simulink model "Integration2022b_May06"  (R2022b)
settings: Solver=FixedStepAuto  StartTime=0.0  StopTime=inf  RelTol=1e-3
model workspace (MAT data in the model file):
  L = 4.165
  SL_ROS_VariableLengthArrays_MaxSizes.CommonInfo.ArrayTruncateAction = 'EmitWarning'
  SL_ROS_VariableLengthArrays_MaxSizes.MsgTypeMap = containers.Map
  SL_ROS_VariableLengthArrays_MaxSizes.MsgTypeMap.serialization.keys = {'example_interfaces/Float64MultiArray', 'std_msgs/Float32MultiArray', 'std_msgs/Float64MultiArray', 'std_msgs/Int32MultiArray'}
  SL_ROS_VariableLengthArrays_MaxSizes.MsgTypeMap.serialization.values{1}.PropertyName = 'data'
  SL_ROS_VariableLengthArrays_MaxSizes.MsgTypeMap.serialization.values{1}.DataType = 'double'
  SL_ROS_VariableLengthArrays_MaxSizes.MsgTypeMap.serialization.values{1}.MaxLength = 3
  SL_ROS_VariableLengthArrays_MaxSizes.MsgTypeMap.serialization.values{2}.PropertyName = 'data'
  SL_ROS_VariableLengthArrays_MaxSizes.MsgTypeMap.serialization.values{2}.DataType = 'single'
  SL_ROS_VariableLengthArrays_MaxSizes.MsgTypeMap.serialization.values{2}.MaxLength = 1260
  SL_ROS_VariableLengthArrays_MaxSizes.MsgTypeMap.serialization.values{3}.PropertyName = 'data'
  SL_ROS_VariableLengthArrays_MaxSizes.MsgTypeMap.serialization.values{3}.DataType = 'double'
  SL_ROS_VariableLengthArrays_MaxSizes.MsgTypeMap.serialization.values{3}.MaxLength = 1386
  SL_ROS_VariableLengthArrays_MaxSizes.MsgTypeMap.serialization.values{4}.PropertyName = 'data'
  SL_ROS_VariableLengthArrays_MaxSizes.MsgTypeMap.serialization.values{4}.DataType = 'int32'
  SL_ROS_VariableLengthArrays_MaxSizes.MsgTypeMap.serialization.values{4}.MaxLength = 3
  SL_ROS_VariableLengthArrays_MaxSizes.MsgTypeMap.serialization.uniformity = 0
  SL_ROS_VariableLengthArrays_MaxSizes.MsgTypeMap.serialization.keyType = 'char'
  SL_ROS_VariableLengthArrays_MaxSizes.MsgTypeMap.serialization.valueType = 'any'
  finalint = 0
  firstWarning = 1
  originalScenarioChecksum = '114339432DE22364D47BB28FC96DC10C'
values from neighbouring files (symbols this model uses):
  D = cross(B-A,C-A)    [HelperCalculateEgoRefPathInfo.m]
  data =     [Part_of_MCity.mat]    (also in curvedroad_Bhanu.mat; plotWPScript.m = [data, [out.x.Data(:, :, i); out.y.Data(:, :, i)]])
  x = [Vertices(Na,1) Vertices(:,1) Vertices(Nb,1)]    [HelperCalculateEgoRefPathInfo.m]    (also in HelperConvertDSPoseToSim3D.m = actor(1).Position(1); xpts.mat = [-29.9023190589 -34.2715935353 -19.4160603154 -19.4160603154)
  y = [Vertices(Na,2) Vertices(:,2) Vertices(Nb,2)]    [HelperCalculateEgoRefPathInfo.m]    (also in HelperConvertDSPoseToSim3D.m = actor(1).Position(2); VehicleOutputFcn.m = [x(1);x(2); x(3); x(4); x(5);x(6)]; ypts.mat = [-62.3254015256 -62.9079714558 -51.8391427821 -48.6350081661)
  z = zeros(1, length(interpX))    [HelperCalculateEgoRefPathInfo.m]
undefined symbols (not defined in the file or in its folder): MinVelocity, WB
libraries: ros2lib x13, mpcsigdimcheck_private x10, robotalgslib x1, mpclib x1, drivingvehiclecontroller x1, slpidlib x1
(part 1 of 5)
settings Model: Creator=akshran  LastModifiedBy=moham
settings DataIOCC: SignalLogging=off  ReturnWorkspaceOutputs=off
settings OptimizationCC: ReuseModelBlockBuffer=on  EnhancedBackFolding=on  PassReuseOutputArgsAs=Individual arguments  ZeroExternalMemoryAtStartup=off  ZeroInternalMemoryAtStartup=off  MaxStackSize=64  OptimizeBlockOrder=speed  DifferentSizesBufferReuse=on  OptimizationCustomize=off  EfficientTunableParamExpr=on
settings DebuggingCC: ParameterTunabilityLossMsg=error  UnconnectedInputMsg=warning  UnconnectedOutputMsg=warning  UnconnectedLineMsg=warning  UnderSpecifiedDimensionMsg=warning
settings HardwareCC: ProdBitPerLong=64  ProdHWDeviceType=AMD->x86-64 (Linux 64)
settings ModelReferenceCC: EnableRefExpFcnMdlSchedulingChecks=on
settings SFSimCC: MATLABDynamicMemAlloc=off
settings RTWCC: Description=Embedded Coder  SystemTargetFile=ert.tlc  HardwareBoard=Robot Operating System 2 (ROS 2)  TLCOptions="-aInlineSetEventsForThisBaseRateFcn=TLC_FALSE -aSuppressMultiTaskScheduler=TLC_FALSE  -aRateBasedStepFcn=0"  TemplateMakefile=ert_default_tmf  Toolchain=Colcon Tools  PortableWordSizes=on  TargetLang=C++  DLArmComputeVersion=19.05
settings CodeAppCC: ForceParamTrailComments=on  IgnoreCustomStorageClasses=off  OperatorAnnotations=on  SimulinkDataObjDesc=on  SFDataObjDesc=on  InsertBlockDesc=on
settings ERTTargetCC: CodeInterfacePackaging=C++ class  RootIOFormat=Structure reference
settings SettingsController: UseSoCProfilerForTargets=0

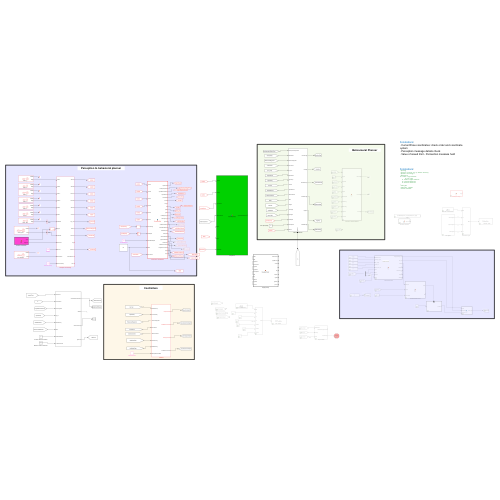
[thumbnail: Simulink's stored preview of the top-level diagram]
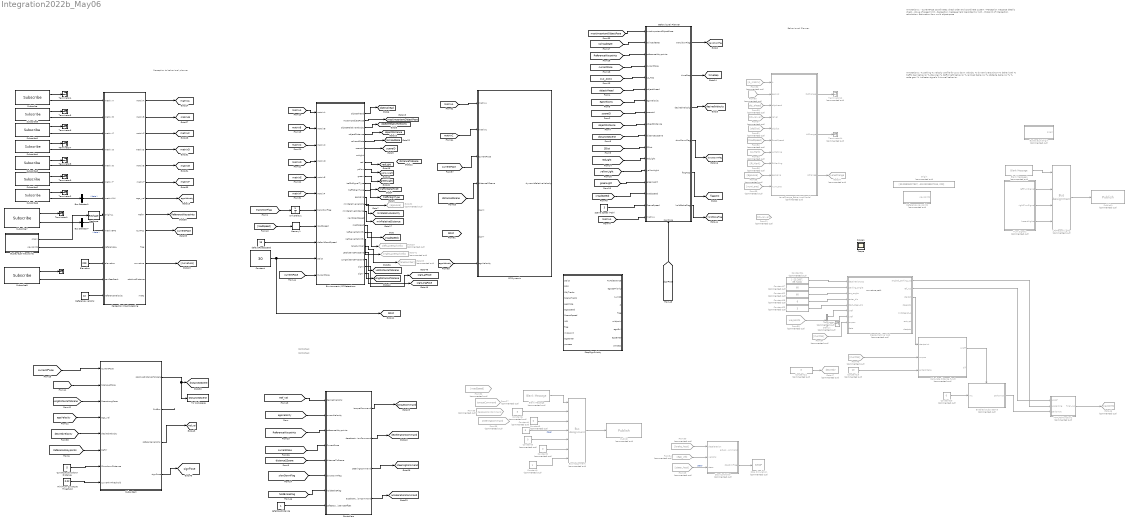
== system Integration2022b_May06 ==
  note: Annotations :
      | - CurrentPose coordinates: check order and coordinate system
      | - Perception message details check
      | - Value of speed limit - Perception message held (persistent or not)
      | - Midpoint of Intersection calculation: Estimation from multi object pose
  note: Behavioural Planner
  note: Perception to behavioral planner
  note: Controllers
  note: Controllers
  note: Annotations :
      | % parking
      | % velocity profile for up & down velocity
      | % dynamic rerouting??
      | % behavioral
      | % traffic sign behavior
      | % stop sign
      | % traffic light behavior
      | % railroad behavior
      | % obstacle behavior
      | %
      | % code gen!
      | % indicator signals
      | % tunnel behavior
  note: curvature path
  " " : Terminator
  Behavioural Planner : Subsystem
      settings: PortSchema="{\"entries\":[{\"content\":{\"sides\":[{\"content\":{\"connectorIds\":[\"In1\",\"In2\",\"In3\",\"In4\",\"In5\",\"In6\",\"In7\",\"In8\",\"In9\",\"In10\",\"In11\",\"In12\",\"In13\",\"In14\",\"In15\",\"In16\",\"In17\"]},\"type\":\"ConnectorPlacement.EquallySpacedRectSide\",\"uuid\":\"494bf481-bdc6-4ab1-b824-5f3bdb3ff01f\"},{\"content\":{\"connectorIds\":[\"Out1\",\"Out2\",\"Out3\",\"Out4\",\"Out5\",\"Out6\"],\"side\":\"RIGHT\"},\"type\":\"ConnectorPlacement.EquallySpacedRectSide\",\"uuid\":\"2468745c-f84f-4a50-a8ff-e7bb2cbe872e\"},{\"content\":{\"side\":\"TOP\"},\"type\":\"ConnectorPlacement.EquallySpacedRectSide\",\"uuid\":\"96280bc7-544f-4b45-a6db-67036c4d07c2\"},{\"content\":{\"connectorIds\":[\"In18\"],\"side\":\"BOTTOM\"},\"type\":\"ConnectorPlacement.EquallySpacedRectSide\",\"uuid\":\"4e16db0f-18f6-4a57-8589-f4480b47e9b5\"}]},\"type\":\"ConnectorPlacement.EquallySpacedConnector\",\"uuid\":\"a6b17eda-b06c-4321-9182-4c70288e8279\"}],\"packageUris\":[\"http://schema.mathworks.com/mf0/Connector/R2020b\"],\"version\":\"1.0\"}"
  Blank Message : ros2lib/Blank Message  Commented=on  messageClass=Message  entityType=std_msgs/Float64MultiArray  messageType=std_msgs/Float64MultiArray  SampleTime=0.01
      settings: LibrarySourceBlock=roslib/ROS 2/Blank Message
  Blank Message1 : ros2lib/Blank Message  Commented=on  messageClass=Message  entityType=geometry_msgs/Vector3  messageType=geometry_msgs/Vector3  SampleTime=0.01
      settings: LibrarySourceBlock=roslib/ROS 2/Blank Message
  BuckeyeLot Origin : MATLAB Function  Commented=on  TreatAsAtomicUnit=on
  BuckeyeLot Waypoints : MATLAB Function  TreatAsAtomicUnit=on
  Bus Assignment : BusAssignment  Commented=on  AssignedSignals=x,y,z,data,data,data
  Bus Selector1 : BusSelector  OutputSignals=data
  Bus Selector7 : BusSelector  OutputSignals=data
  Calculate distance func3 : MATLAB Function  Commented=on  TreatAsAtomicUnit=on
  Constant : Constant  Value=30
  Constant1 : Constant  Commented=on
  Constant17 : Constant  Commented=on  Value=60
  Constant18 : Constant  Commented=on  Value=6
  Constant19 : Constant  Commented=on  Value=10
  Constant{2..3,5,20} (4 alike) : Constant  Commented=on  Value=0
  Constant21 : Constant  Commented=on  Value=3
  Constant22 : Constant  Commented=on  Value=60
  Constant23 : Constant  Commented=on  Value=3
  Constant24 : Constant  Commented=on  Value=[ -25.2607, 39.7402]
  Constant4 : Constant  Commented=on  Value=5
  Constant6 : Constant  Commented=on  Value=5
  Controllers : Subsystem
  Create Parking Wp2 : MATLAB Function  Commented=on  TreatAsAtomicUnit=on
  Curvature Slowdown Distance : Constant  Value=5
  Demux : Demux  Commented=on  Outputs=3
  Elevation : Constant  Value=229
  Enabled Subsystem3 : Subsystem  Commented=on  TreatAsAtomicUnit=on
  Environment / SF Detections : MATLAB Function  TreatAsAtomicUnit=on
  From11 : From  Commented=on  GotoTag=obj_rel_vel  TagVisibility=global
  From27 : From  Commented=on  GotoTag=torqueCommand  TagVisibility=global
  From29 : From  Commented=on  GotoTag=steer_host  TagVisibility=global
  From30 : From  Commented=on  GotoTag=brake_host  TagVisibility=global
  From32 : From  Commented=on  GotoTag=roadSpeed
  From34 : From  Commented=on  GotoTag=ego_vel  TagVisibility=global
  From35 : From  Commented=on  GotoTag=decelerationCommand  TagVisibility=global
  From36 : From  Commented=on  GotoTag=steeringCommand  TagVisibility=global
  From37 : From  Commented=on  GotoTag=obj_rel_vel  TagVisibility=global
  From39 : From  Commented=on  GotoTag=obj_ahead  TagVisibility=global
  From49 : From  Commented=on  GotoTag=CurrPos
  From50 : From  Commented=on  GotoTag=A_matrix
  From51 : From  Commented=on  GotoTag=objDist  TagVisibility=global
  From52 : From  Commented=on  GotoTag=RoadSpeed
  From53 : From  Commented=on  GotoTag=LLMark
  From54 : From  Commented=on  GotoTag=CurrPos
  From55 : From  Commented=on  GotoTag=waypoints  TagVisibility=global
  From56 : From  Commented=on  GotoTag=RLMark
  From58 : From  Commented=on  GotoTag=EgoLane
  From59 : From  Commented=on  GotoTag=numLane
  From60 : From  Commented=on  GotoTag=ego_vel  TagVisibility=global
  Goto29 : Goto  Commented=on  GotoTag=leftLaneMarkInfo
  Goto32 : Goto  Commented=on  GotoTag=egoLane
  Goto35 : Goto  Commented=on  GotoTag=laneNumber
  Goto37 : Goto  Commented=on  GotoTag=LaneChange  TagVisibility=global
  Goto41 : Goto  Commented=on  GotoTag=rightLaneMarkInfo
  Goto46 : Goto  Commented=on  GotoTag=waypoints  TagVisibility=global
  Goto47 : Goto  Commented=on  GotoTag=desiredV  TagVisibility=global
  L/R/Hazard Lights : BusAssignment  Commented=on  AssignedSignals=x,y,z
  LaneChange_BehavioralModel : MATLAB Function  Commented=on  TreatAsAtomicUnit=on
  MATLAB Function2 : MATLAB Function  Commented=on  TreatAsAtomicUnit=on
  Memory1 : Memory  InitialCondition=15
  "Minimum Curvature Threshold " : Constant  Value=0.02
  Origin : Constant  Commented=on  Value=[39.99806227837, -83.03238507155, 229]
  Perception Pre-Processing : Subsystem
  Publish : ros2lib/Publish  Commented=on  topicSource=Select from ROS network  topic=/can_forward  messageType=geometry_msgs/Vector3  QOSHistory=Keep last  QOSDepth=1  QOSReliability=Reliable  QOSDurability=Volatile
      settings: LibrarySourceBlock=roslib/ROS 2/Publish
  Publish1 : ros2lib/Publish  Commented=on  topicSource=Specify your own  topic=/indicator_lights  messageType=geometry_msgs/Vector3  QOSHistory=Keep last  QOSDepth=1  QOSReliability=Reliable  QOSDurability=Volatile
      settings: LibrarySourceBlock=roslib/ROS 2/Publish
  Reference velocity : Constant  Value=10
  Reference waypoints : MATLAB Function  Commented=on  TreatAsAtomicUnit=on
  Reshape : Reshape  OutputDimensionality=Row vector (2-D)
  SF Dynamic : MATLAB Function  TreatAsAtomicUnit=on
  Scene Speed (Mph) : Constant  Value=3
  Stop Controller : Subsystem  Commented=on
  Stop Simulation : Stop  Commented=on
  StopSignPriority : MATLAB Function  TreatAsAtomicUnit=on
  Subscribe : ros2lib/Subscribe  topicSource=Select from ROS network  topic=/matrix_A  messageType=std_msgs/Float64MultiArray  sampleTime=-1  QOSHistory=Keep last  QOSDepth=1  QOSReliability=Reliable  QOSDurability=Volatile
      settings: LibrarySourceBlock=roslib/ROS 2/Subscribe
  Subscribe1 : ros2lib/Subscribe  topicSource=Select from ROS network  topic=/matrix_C  messageType=std_msgs/Float64MultiArray  sampleTime=-1  QOSHistory=Keep last  QOSDepth=1  QOSReliability=Reliable  QOSDurability=Volatile
      settings: LibrarySourceBlock=roslib/ROS 2/Subscribe
  Subscribe2 : ros2lib/Subscribe  topicSource=Select from ROS network  topic=/matrix_F  messageType=std_msgs/Float64MultiArray  sampleTime=-1  QOSHistory=Keep last  QOSDepth=1  QOSReliability=Reliable  QOSDurability=Volatile
      settings: LibrarySourceBlock=roslib/ROS 2/Subscribe
  Subscribe3 : ros2lib/Subscribe  topicSource=Select from ROS network  topic=/matrix_E  messageType=std_msgs/Float64MultiArray  sampleTime=-1  QOSHistory=Keep last  QOSDepth=1  QOSReliability=Reliable  QOSDurability=Volatile
      settings: LibrarySourceBlock=roslib/ROS 2/Subscribe
  Subscribe4 : ros2lib/Subscribe  topicSource=Select from ROS network  topic=/matrix_D  messageType=std_msgs/Float64MultiArray  sampleTime=-1  QOSHistory=Keep last  QOSDepth=1  QOSReliability=Reliable  QOSDurability=Volatile
      settings: LibrarySourceBlock=roslib/ROS 2/Subscribe
  Subscribe5 : ros2lib/Subscribe  topicSource=Select from ROS network  topic=/matrix_B  messageType=std_msgs/Float64MultiArray  sampleTime=-1  QOSHistory=Keep last  QOSDepth=1  QOSReliability=Reliable  QOSDurability=Volatile
      settings: LibrarySourceBlock=roslib/ROS 2/Subscribe
  Subscribe6 : ros2lib/Subscribe  topicSource=Select from ROS network  topic=/matrix_IMU  messageType=std_msgs/Float64MultiArray  sampleTime=-1  QOSHistory=Keep all  QOSDepth=1  QOSReliability=Reliable  QOSDurability=Volatile
      settings: LibrarySourceBlock=roslib/ROS 2/Subscribe
  Subscribe7 : ros2lib/Subscribe  topicSource=Specify your own  topic=/matrix_GPS  messageType=std_msgs/Float64MultiArray  sampleTime=-1  QOSHistory=Keep all  QOSDepth=1  QOSReliability=Reliable  QOSDurability=Volatile
      settings: LibrarySourceBlock=roslib/ROS 2/Subscribe
  Subscribe9 : ros2lib/Subscribe  topicSource=Specify your own  topic=/can_feedback  messageType=geometry_msgs/Vector3  sampleTime=-1  QOSHistory=Keep all  QOSDepth=1  QOSReliability=Reliable  QOSDurability=Volatile
      settings: LibrarySourceBlock=roslib/ROS 2/Subscribe
  Subsystem : Subsystem
  Terminator : Terminator  Commented=on
  Terminator{1..2,4..9} (8 alike) : Terminator
  Terminator12 : Terminator  Commented=on
  Terminator14 : Terminator  Commented=on
  To Workspace : ToWorkspace  VariableName=Distance2Scene  SaveFormat=Structure With Time  SampleTime=-1
  Turn Signals : Subsystem  Commented=on
  Unit Delay1 : UnitDelay  SampleTime=0.01  HasFrameUpgradeWarning=on
  defaultRoadSpeed : Constant  Value=15
  safeStopDistance : Constant
  Scope : Scope
  Scope1 : Scope
  tag scope: LatDistanceToScene=global, LongDistanceToScene=global, Ref_Vel=global, ReferenceWaypoints=global, SDist=global, accelerationCommand=global, currentPose=global, decelerationCommand=global, desiredVelocity=global, distance2Scene=global, distanceToScene=global, egoVelocity=global, flagACC=global, greenLight=global, holdBrakeFlag=global, matrixA=global, matrixB=global, matrixC=global, matrixD=global, matrixE=global, matrixF=global, minRelativeDistance=global, minRelativeVelocity=global, mostImportantObjectPose=global, objectAhead=global, objectDistance=global, objectRelativeVelocity=global, railroadGate=global, redLight=global, sceneID=global, signLatPose=global, signLongPose=global, signPose=global, slowDownFlag=global, steeringCommand=global, timeGap=global, torqueCommand=global, trafficSignType=global, trafficSignalType=global, transitionFlag=global, yellowLight=global
  wires:
  [transitionFlag] -> Unit Delay1/1
  [objectAhead] -> Behavioural Planner/6(objectAhead)
  [egoVelocity] -> Behavioural Planner/7(egoVelocity)
  [objectDistance] -> Behavioural Planner/9(objectDistance)
  [SDist] -> Behavioural Planner/11(SDist)
  Behavioural Planner/5(flagACC) -> [flagACC]
  Behavioural Planner/1(transitionFlag) -> [transitionFlag]
  Behavioural Planner/2(timeGap) -> [timeGap]
  Behavioural Planner/3(desiredVelocity) -> [desiredVelocity]
  Behavioural Planner/4(slowDownFlag) -> [slowDownFlag]
  [LC_ACC] -> Behavioural Planner/5(LC_ACC)
  [redLight] -> Behavioural Planner/12(redLight)
  [yellowLight] -> Behavioural Planner/13(yellowLight)
  [greenLight] -> Behavioural Planner/14(greenLight)
  [railroadGate] -> Behavioural Planner/2(railroadGate)
  [currentPose] -> Behavioural Planner/4(currentPose)
  From50/1 -> LaneChange_BehavioralModel/1(A)
  From39/1 -> LaneChange_BehavioralModel/3(objahead)
  From37/1 -> LaneChange_BehavioralModel/4(relvel)
  From51/1 -> LaneChange_BehavioralModel/5(objdist)
  From52/1 -> LaneChange_BehavioralModel/6(RoadSpeed)
  From53/1 -> LaneChange_BehavioralModel/7(LLMarking)
  From56/1 -> LaneChange_BehavioralModel/8(RLMarking)
  From58/1 -> LaneChange_BehavioralModel/9(egoLane)
  From59/1 -> LaneChange_BehavioralModel/10(numLane)
  From60/1 -> LaneChange_BehavioralModel/2(egovel)
  LaneChange_BehavioralModel/1(RLChange) -> Terminator12/1
  LaneChange_BehavioralModel/2(LLChange) -> Terminator14/1
  LaneChange_BehavioralModel/3(LChange) -> Goto37/1
  Subscribe2/1 -> Terminator9/1
  Subscribe5/1 -> Terminator5/1
  Subscribe1/1 -> Terminator6/1
  Subscribe3/1 -> Terminator8/1
  Subscribe/1 -> Terminator4/1
  Subscribe4/1 -> Terminator7/1
  Subscribe9/1 -> " "/1
  Perception Pre-Processing/6(matrixF) -> [matrixF]
  Perception Pre-Processing/4(matrixD) -> [matrixD]
  Perception Pre-Processing/1(matrixA) -> [matrixA]
  Perception Pre-Processing/2(matrixB) -> [matrixB]
  Subscribe/2 -> Perception Pre-Processing/1(matrix A)
  Subscribe5/2 -> Perception Pre-Processing/2(matrix B)
  Subscribe1/2 -> Perception Pre-Processing/3(matrix C)
  Subscribe4/2 -> Perception Pre-Processing/4(matrix D)
  Subscribe3/2 -> Perception Pre-Processing/5(matrix E)
  Subscribe2/2 -> Perception Pre-Processing/6(matrix F)
  BuckeyeLot Waypoints/1(origin) -> Reshape/1
  BuckeyeLot Waypoints/2(waypoints) -> Perception Pre-Processing/10(referenceLL)
  Elevation/1 -> Perception Pre-Processing/11(elevation)
  Subscribe9/2 -> Perception Pre-Processing/12(canFeedback)
  Reference velocity/1 -> Perception Pre-Processing/13(referenceVelocity)
  Perception Pre-Processing/7(ego_vel) -> [egoVelocity]
  Perception Pre-Processing/8(RefXY) -> [ReferenceWaypoints]
  Perception Pre-Processing/9(CurrPos) -> [currentPose]
  Perception Pre-Processing/11(curvature) -> [curvature]
  Perception Pre-Processing/3(matrixC) -> [matrixC]
  [matrixA] -> Environment / SF Detections/1(matrixA)
  [matrixB] -> Environment / SF Detections/2(matrixB)
  [matrixC] -> Environment / SF Detections/3(matrixC)
  [matrixD] -> Environment / SF Detections/4(matrixD)
  [matrixE] -> Environment / SF Detections/5(matrixE)
  Unit Delay1/1 -> Environment / SF Detections/7(transitionFlag)
  Constant/1 -> [SDist], Environment / SF Detections/10(SDist)
  Controllers/4(accelerationCommand) -> [accelerationCommand]
  Controllers/1(torqueCommand) -> [torqueCommand]
  Controllers/3(steeringCommand) -> [steeringCommand]
  [ReferenceWaypoints] -> Controllers/3(referenceWaypoints)
  [currentPose] -> Controllers/4(CurrentPose)
  [egoVelocity] -> Controllers/2(currentVelocity)
  Controllers/2(decelerationCommand) -> [decelerationCommand]
  [slowDownFlag] -> Controllers/6(slowDownFlag)
  Bus Assignment/1 -> Publish/1
  Constant6/1 -> Bus Assignment/2
  Blank Message/1 -> Bus Assignment/1
  Constant5/1 -> Bus Assignment/3
  From30/1 -> Stop Controller/1(deceleration)
  From34/1 -> Stop Controller/2(velocity)
  From29/1 -> Stop Controller/3(steer)  "steer"
  Stop Controller/2(stopSimFlag) -> Stop Simulation/1
  Turn Signals/1(leftTurnSignal) -> L/R/Hazard Lights/2
  Turn Signals/3(hazardLights) -> L/R/Hazard Lights/4
  Turn Signals/2(rightTurnSignal) -> L/R/Hazard Lights/3
  L/R/Hazard Lights/1 -> Publish1/1
  Blank Message1/1 -> L/R/Hazard Lights/1
  [ReferenceWaypoints] -> Behavioural Planner/3(referenceWaypoints)
  Environment / SF Detections/1(objectAhead) -> [objectAhead]
  Environment / SF Detections/2(mostImpObjectPose) -> [mostImportantObjectPose]
  Environment / SF Detections/3(objectRelativeVelocity) -> [objectRelativeVelocity]
  Environment / SF Detections/4(objectDistance) -> [objectDistance]
  Environment / SF Detections/5(railroadGate) -> [railroadGate]
  Environment / SF Detections/6(sceneId) -> [sceneID]
  Environment / SF Detections/8(red) -> [redLight]
  Environment / SF Detections/9(yellow) -> [yellowLight]
  Environment / SF Detections/10(green) -> [greenLight]
  Environment / SF Detections/11(trafficSignalType) -> [trafficSignalType]
  Environment / SF Detections/12(trafficSignType) -> [trafficSignType]
  Environment / SF Detections/13(egoLane) -> Goto32/1
  Environment / SF Detections/14(minRelativeVelocity) -> [minRelativeVelocity]
  Environment / SF Detections/15(minRelativeDistance) -> [minRelativeDistance]
  Environment / SF Detections/20(laneNumber) -> Goto35/1
  Environment / SF Detections/18(leftLaneMarkInfo) -> Goto29/1
  Environment / SF Detections/19(rightLaneMarkInfo) -> Goto41/1
  [matrixF] -> Environment / SF Detections/6(matrixF)
  safeStopDistance/1 -> Controllers/8(safeStopDistanceOffset)
  Scene Speed (Mph)/1 -> Behavioural Planner/16(SceneSpeed)
  Environment / SF Detections/17(roadSpeed) -> [roadSpeed]
  [mostImportantObjectPose] -> Behavioural Planner/1(mostImportantObjectPose)
  Reshape/1 -> Perception Pre-Processing/8(originLL)
  Subscribe7/2 -> Bus Selector7/1
  Bus Selector7/1 -> Perception Pre-Processing/9(matrixGPS)  "<data>"
  Bus Selector1/1 -> Perception Pre-Processing/7(matrixIMU)  "<data>"
  Subscribe7/1 -> Terminator1/1
  Subscribe6/1 -> Terminator2/1
  Subscribe6/2 -> Bus Selector1/1
  [distance2Scene] -> Behavioural Planner/10(distance2Scene)
  [distance2Scene] -> Controllers/5(distanceToScene)
  Constant4/1 -> Bus Assignment/4  "steer"
  [sceneID] -> Behavioural Planner/8(sceneId)
  [egoVelocity] -> Subsystem/4(ego_vel)
  [desiredVelocity] -> Subsystem/5(desiredVelocity)
  [ReferenceWaypoints] -> Subsystem/6(RefXY)
  Curvature Slowdown Distance/1 -> Subsystem/7(SlowdownDistance)
  "Minimum Curvature Threshold "/1 -> Subsystem/8(curveMinThreshold)
  Subsystem/1(relativeDistanceToScene) -> To Workspace/1, [distance2Scene]
  [currentPose] -> Subsystem/1(CurrentPose)
  Environment / SF Detections/21(LatDistanceToScene) -> [LatDistanceToScene]
  Environment / SF Detections/22(LongDistanceToScene) -> [LongDistanceToScene]
  [LatDistanceToScene] -> Subsystem/2(SceneLatPose)
  [LongDistanceToScene] -> Subsystem/3(SceneLongPose)
  Subsystem/3(referenceVelocity) -> [Ref_Vel]
  [Ref_Vel] -> Controllers/1(desiredVelocity)
  Perception Pre-Processing/5(matrixE) -> [matrixE]
  [currentPose] -> Environment / SF Detections/11(CurrentPose)
  [roadSpeed] -> Behavioural Planner/15(roadSpeed)
  Behavioural Planner/6(holdBrakeFlag) -> [holdBrakeFlag]
  [holdBrakeFlag] -> Controllers/7(holdBrakeFlag)
  [matrixA] -> Behavioural Planner/17(matrixA)
  [signPose] -> Behavioural Planner/18(signPose)
  Subsystem/4(signPose) -> [signPose]
  defaultRoadSpeed/1 -> Environment / SF Detections/9(defaultRoadSpeed)
  Constant20/1 -> Enabled Subsystem3/1(In1)
  Constant18/1 -> Create Parking Wp2/4(enter_dis)
  Create Parking Wp2/2(ref_wp) -> MATLAB Function2/1(wpref)
  Constant19/1 -> Calculate distance func3/3(entercriteria)
  Constant23/1 -> Create Parking Wp2/5(start_steer_dis)
  From49/1 -> Calculate distance func3/2(curpos)
  Constant17/1 -> Create Parking Wp2/2(parking_angle)
  Calculate distance func3/1(onoff) -> Enabled Subsystem3/Enable
  Constant22/1 -> Create Parking Wp2/3(arc_angle)
  Constant21/1 -> Goto47/1
  Enabled Subsystem3/1(parkornot) -> MATLAB Function2/3(parkornot)
  Constant24/1 -> Create Parking Wp2/1(destinationpos)
  Create Parking Wp2/1(angled_parking_wp) -> MATLAB Function2/2(wpparking)
  MATLAB Function2/1(final_wp) -> Goto46/1
  Create Parking Wp2/3(startpt) -> Calculate distance func3/1(startpoint)
  From54/1 -> Create Parking Wp2/8(curpos)
  From55/1 -> Demux/1
  Demux/1 -> Create Parking Wp2/6(xref)
  Demux/2 -> Create Parking Wp2/7(yref)
  Demux/3 -> Terminator/1
  Constant1/1 -> Bus Assignment/7
  Constant2/1 -> Bus Assignment/6
  Constant3/1 -> Bus Assignment/5
  [roadSpeed] -> Memory1/1
  Memory1/1 -> Environment / SF Detections/8("roadSpeed ")
  [currentPose] -> SF Dynamic/3(CurrentPose)
  [matrixA] -> SF Dynamic/1(matrixA)
  [distance2Scene] -> SF Dynamic/4(distance2Scene)
  Subsystem/2(OutBus) -> ?
  [matrixC] -> SF Dynamic/2(matrixC)
  Environment / SF Detections/23(signX) -> [signLatPose]
  Environment / SF Detections/24(signY) -> [signLongPose]
  [egoVelocity] -> SF Dynamic/7(egoVelocity)

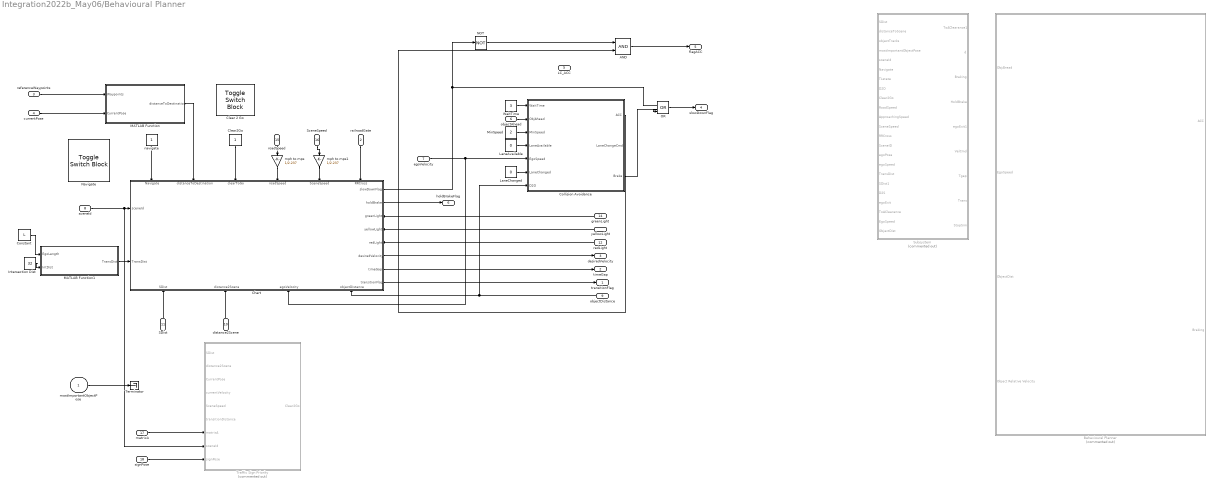
== system Integration2022b_May06/Behavioural Planner ==
  mostImportantObjectPose : Inport
  railroadGate : Inport  Port=2
  referenceWaypoints : Inport  Port=3
  currentPose : Inport  Port=4
  LC_ACC : Inport  Port=5
  objectAhead : Inport  Port=6
  egoVelocity : Inport  Port=7
  sceneId : Inport  Port=8
  objectDistance : Inport  Port=9
  distance2Scene : Inport  Port=10
  SDist : Inport  Port=11
  redLight : Inport  Port=12
  yellowLight : Inport  Port=13
  greenLight : Inport  Port=14
  roadSpeed : Inport  Port=15
  SceneSpeed : Inport  Port=16
  matrixA : Inport  Port=17
  signPose : Inport  Port=18
  AND : Logic  IconShape=distinctive  AllPortsSameDT=off  OutDataTypeStr=fixdt(1,16)
  Behavioural Planner : Subsystem  Commented=on
  Chart : Stateflow chart  TreatAsAtomicUnit=on
      settings: PortSchema="{\"entries\":[{\"content\":{\"sides\":[{\"content\":{\"connectorIds\":[\"In14\",\"In4\"]},\"type\":\"ConnectorPlacement.EquallySpacedRectSide\",\"uuid\":\"81aca70f-0947-49fb-b60a-be241e44193b\"},{\"content\":{\"connectorIds\":[\"Out4\",\"Out5\",\"In1\",\"In2\",\"In3\",\"Out1\",\"Out2\",\"Out3\"],\"side\":\"RIGHT\"},\"type\":\"ConnectorPlacement.EquallySpacedRectSide\",\"uuid\":\"e7b9645e-3711-4964-ac9b-0199dd335e99\"},{\"content\":{\"connectorIds\":[\"In15\",\"In11\",\"In12\",\"In13\",\"In7\",\"In9\"],\"side\":\"TOP\"},\"type\":\"ConnectorPlacement.EquallySpacedRectSide\",\"uuid\":\"6876f024-944b-4540-9404-d68f37763657\"},{\"content\":{\"connectorIds\":[\"In8\",\"In10\",\"In5\",\"In6\"],\"side\":\"BOTTOM\"},\"type\":\"ConnectorPlacement.EquallySpacedRectSide\",\"uuid\":\"44acab73-cdde-4edf-95df-27422644ccab\"}]},\"type\":\"ConnectorPlacement.EquallySpacedConnector\",\"uuid\":\"d2c31c01-e447-43db-8d2b-8b98a0ca291a\"}],\"packageUris\":[\"http://schema.mathworks.com/mf0/Connector/R2020b\"],\"version\":\"1.0\"}"
  Clear 2 Go : ToggleSwitchBlock
      settings: Values={{'Off', 'On'}, [0 1]}
  Clear2Go : Constant
  Collision Avoidance : Stateflow chart  TreatAsAtomicUnit=on
  Constant : Constant  Value=L
  Intersection Dist : Constant  Value=32
  LaneAvailable : Constant  Value=0
  LaneChanged : Constant  Value=0
  MATLAB Function : MATLAB Function  TreatAsAtomicUnit=on
  MATLAB Function1 : MATLAB Function  TreatAsAtomicUnit=on
  MinSpeed : Constant  Value=2
  NOT : Logic  Operator=NOT  IconShape=distinctive  AllPortsSameDT=off  OutDataTypeStr=boolean
  Navigate : ToggleSwitchBlock
      settings: Values={{'Off', 'On'}, [0 1]}
  OR : Logic  Operator=OR  IconShape=distinctive  AllPortsSameDT=off  OutDataTypeStr=boolean
  Subsystem : Subsystem  Commented=on
  Terminator : Terminator
  Traffic Sign Priority : MATLAB Function  Commented=on  TreatAsAtomicUnit=on
  WaitTime : Constant  Value=3
  mph to mps : Gain  Gain=1/2.237
  mph to mps1 : Gain  Gain=1/2.237
  navigate : Constant
  transitionFlag : Outport
  timeGap : Outport  Port=2
  desiredVelocity : Outport  Port=3
  slowDownFlag : Outport  Port=4
  flagACC : Outport  Port=5
  holdBrakeFlag : Outport  Port=6
  wires:
  Clear2Go/1 -> Chart/12(clearToGo)
  objectDistance/1 -> Collision Avoidance/7(D2O), Chart/6(objectDistance)
  WaitTime/1 -> Collision Avoidance/1(WaitTime)
  navigate/1 -> Chart/15(Navigate)
  egoVelocity/1 -> Collision Avoidance/5(EgoSpeed), Chart/5(egoVelocity)
  LaneAvailable/1 -> Collision Avoidance/4(LaneAvailable)
  currentPose/1 -> MATLAB Function/2(CurrentPose)
  MinSpeed/1 -> Collision Avoidance/3(MinSpeed)
  LaneChanged/1 -> Collision Avoidance/6(LaneChanged)
  objectAhead/1 -> Collision Avoidance/2(ObjAhead)
  MATLAB Function/1(distanceToDestination) -> Chart/11(distanceToDestination)
  Chart/3(transitionFlag) -> transitionFlag/1
  Chart/1(desiredVelocity) -> desiredVelocity/1
  SDist/1 -> Chart/8(SDist)
  distance2Scene/1 -> Chart/10(distance2Scene)
  Chart/2(timeGap) -> timeGap/1
  Collision Avoidance/1(ACC) -> AND/2
  NOT/1 -> AND/1
  Chart/4(slowDownFlag) -> NOT/1, OR/1
  OR/1 -> slowDownFlag/1
  Collision Avoidance/3(Brake) -> OR/2
  Constant/1 -> MATLAB Function1/1(EgoLength)
  Intersection Dist/1 -> MATLAB Function1/2(IntDist)
  MATLAB Function1/1(TransDist) -> Chart/4(TransDist)
  yellowLight/1 -> Chart/2(yellowLight)
  redLight/1 -> Chart/3(redLight)
  railroadGate/1 -> Chart/9(RRCross)
  referenceWaypoints/1 -> MATLAB Function/1(Waypoints)
  mph to mps/1 -> Chart/13(roadSpeed)
  roadSpeed/1 -> mph to mps/1
  greenLight/1 -> Chart/1(greenLight)
  AND/1 -> flagACC/1
  SceneSpeed/1 -> mph to mps1/1
  mph to mps1/1 -> Chart/7(SceneSpeed)
  mostImportantObjectPose/1 -> Terminator/1
  Chart/5(holdBrake) -> holdBrakeFlag/1
  matrixA/1 -> Traffic Sign Priority/7(matrixA)
  signPose/1 -> Traffic Sign Priority/9(signPose)
  sceneId/1 -> Traffic Sign Priority/8(sceneId), Chart/14(sceneId)

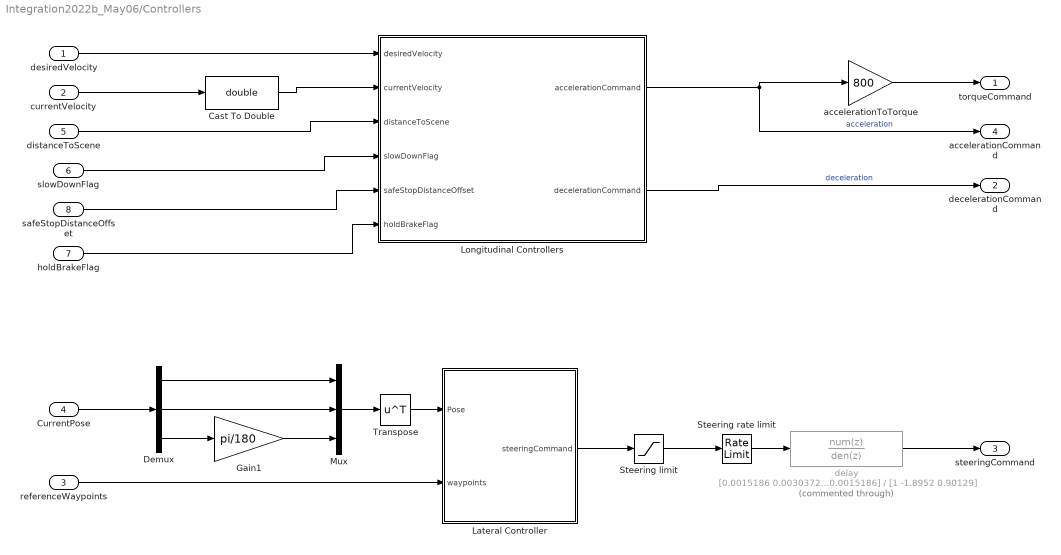
== system Integration2022b_May06/Controllers ==
  desiredVelocity : Inport
  currentVelocity : Inport  Port=2
  referenceWaypoints : Inport  Port=3
  CurrentPose : Inport  Port=4
  distanceToScene : Inport  Port=5
  slowDownFlag : Inport  Port=6
  holdBrakeFlag : Inport  Port=7
  safeStopDistanceOffset : Inport  Port=8
  Cast To Double : DataTypeConversion  OutDataTypeStr=double  SaturateOnIntegerOverflow=off  RndMeth=Floor
  Demux : Demux  Outputs=3
  Gain1 : Gain  Gain=pi/180
  Lateral Controller : Subsystem
  Longitudinal Controllers : Subsystem
  Mux : Mux  Inputs=3
  Steering limit : Saturate  UpperLimit=540  LowerLimit=-540  LinearizeAsGain=off
  Steering rate limit : RateLimiter  RisingSlewLimit=600  FallingSlewLimit=-600  SampleTimeMode=inherited
  Transpose : Math  Operator=transpose  SignedPower=on
  accelerationToTorque : Gain  Gain=800
  delay : DiscreteTransferFcn  Commented=through  Numerator=[0.0015186 0.0030372 0.0015186]  Denominator=[1 -1.8952 0.90129]  SampleTime=0.01
  torqueCommand : Outport
  decelerationCommand : Outport  Port=2
  steeringCommand : Outport  Port=3
  accelerationCommand : Outport  Port=4
  wires:
  desiredVelocity/1 -> Longitudinal Controllers/1(desiredVelocity)
  Longitudinal Controllers/2(decelerationCommand) -> decelerationCommand/1  "deceleration"
  Longitudinal Controllers/1(accelerationCommand) -> accelerationToTorque/1, accelerationCommand/1  "acceleration"
  currentVelocity/1 -> Cast To Double/1
  CurrentPose/1 -> Demux/1
  referenceWaypoints/1 -> Lateral Controller/2(waypoints)
  Cast To Double/1 -> Longitudinal Controllers/2(currentVelocity)
  Steering limit/1 -> Steering rate limit/1
  Lateral Controller/1(steeringCommand) -> Steering limit/1
  delay/1 -> steeringCommand/1
  accelerationToTorque/1 -> torqueCommand/1
  distanceToScene/1 -> Longitudinal Controllers/3(distanceToScene)
  slowDownFlag/1 -> Longitudinal Controllers/4(slowDownFlag)
  Mux/1 -> Transpose/1
  Demux/3 -> Gain1/1
  Demux/2 -> Mux/2
  Demux/1 -> Mux/1
  Transpose/1 -> Lateral Controller/1(Pose)
  Gain1/1 -> Mux/3
  safeStopDistanceOffset/1 -> Longitudinal Controllers/5(safeStopDistanceOffset)
  Steering rate limit/1 -> delay/1
  holdBrakeFlag/1 -> Longitudinal Controllers/6(holdBrakeFlag)

== system Integration2022b_May06/Enabled Subsystem3 ==
  In1 : Inport
  Enable : EnablePort
  Constant : Constant
  Sum : Sum
  parkornot : Outport
  wires:
  In1/1 -> Sum/1
  Constant/1 -> Sum/2
  Sum/1 -> parkornot/1

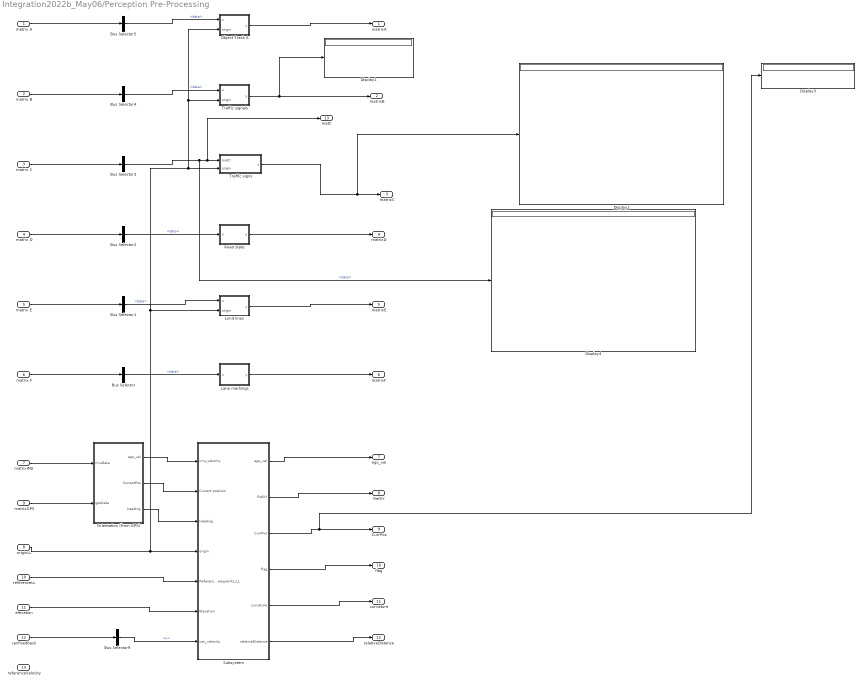
== system Integration2022b_May06/Perception Pre-Processing ==
  matrix A : Inport
  matrix B : Inport  Port=2
  matrix C : Inport  Port=3
  matrix D : Inport  Port=4
  matrix E : Inport  Port=5
  matrix F : Inport  Port=6
  matrixIMU : Inport  Port=7
  originLL : Inport  Port=8
  matrixGPS : Inport  Port=9
  referenceLL : Inport  Port=10
  elevation : Inport  Port=11
  canFeedback : Inport  Port=12
  referenceVelocity : Inport  Port=13
  Bus Selector{,1..5} (6 alike) : BusSelector  OutputSignals=data
  Bus Selector9 : BusSelector  OutputSignals=x
  Display{1..4} (4 alike) : Display
  Lane markings : MATLAB Function  TreatAsAtomicUnit=on
  Limit lines : MATLAB Function  TreatAsAtomicUnit=on
  Object Track A : MATLAB Function  TreatAsAtomicUnit=on
  Orientation (from GPS) : MATLAB Function  TreatAsAtomicUnit=on
  Road state : MATLAB Function  TreatAsAtomicUnit=on
  Subsystem : Subsystem
  Traffic signals : MATLAB Function  TreatAsAtomicUnit=on
  Traffic signs : MATLAB Function  TreatAsAtomicUnit=on
  matrixA : Outport
  matrixB : Outport  Port=2
  matrixC : Outport  Port=3
  matrixD : Outport  Port=4
  matrixE : Outport  Port=5
  matrixF : Outport  Port=6
  ego_vel : Outport  Port=7
  RefXY : Outport  Port=8
  CurrPos : Outport  Port=9
  flag : Outport  Port=10
  curvature : Outport  Port=11
  relativeDistance : Outport  Port=12
  matC : Outport  Port=13
  wires:
  Bus Selector2/1 -> Road state/1(u)  "<data>"
  matrixIMU/1 -> Orientation (from GPS)/1(imuData)
  Bus Selector1/1 -> Limit lines/1(u)  "<data>"
  Bus Selector4/1 -> Traffic signals/1(u)  "<data>"
  Bus Selector9/1 -> Subsystem/7(can_velocity)  "<x>"
  Bus Selector5/1 -> Object Track A/1(u)  "<data>"
  Orientation (from GPS)/1(ego_vel) -> Subsystem/1(imu_velocity)
  Road state/1(y) -> matrixD/1
  matrix A/1 -> Bus Selector5/1
  Bus Selector3/1 -> Display4/1, matC/1, Traffic signs/1(matC)  "<data>"
  matrix E/1 -> Bus Selector1/1
  Bus Selector/1 -> Lane markings/1(u)  "<data>"
  Orientation (from GPS)/2(CurrentPos) -> Subsystem/2(Current position)
  Limit lines/1(y) -> matrixE/1
  Orientation (from GPS)/3(heading) -> Subsystem/3(Heading)
  Object Track A/1(y) -> matrixA/1
  matrix D/1 -> Bus Selector2/1
  matrix C/1 -> Bus Selector3/1
  matrix B/1 -> Bus Selector4/1
  Subsystem/4(flag) -> flag/1
  matrix F/1 -> Bus Selector/1
  canFeedback/1 -> Bus Selector9/1
  referenceLL/1 -> Subsystem/5(Reference_waypoints_LL)
  elevation/1 -> Subsystem/6(Elevation)
  Subsystem/3(CurrPos) -> CurrPos/1, Display3/1
  Subsystem/1(ego_vel) -> ego_vel/1
  Lane markings/1(y) -> matrixF/1
  Subsystem/2(RefXY) -> RefXY/1
  Subsystem/5(curvature) -> curvature/1
  matrixGPS/1 -> Orientation (from GPS)/2(gpsData)
  Subsystem/6(relativeDistance) -> relativeDistance/1
  originLL/1 -> Limit lines/2(origin), Object Track A/2(origin), Traffic signals/2(origin), Traffic signs/2(origin), Subsystem/4(origin)
  Traffic signals/1(y) -> Display1/1, matrixB/1
  Traffic signs/1(y) -> Display2/1, matrixC/1

== system Integration2022b_May06/Stop Controller ==
  deceleration : Inport
  velocity : Inport  Port=2
  steer : Inport  Port=3
  Brake Safety : MATLAB Function  TreatAsAtomicUnit=on
  MATLAB Function5 : MATLAB Function  TreatAsAtomicUnit=on
  Steer Safety : MATLAB Function  TreatAsAtomicUnit=on
  actualSteeringCommand : Outport
  stopSimFlag : Outport  Port=2
  wires:
  Brake Safety/1(actualDeceleration) -> MATLAB Function5/2(braking)
  [accelerationCommand] -> MATLAB Function5/1(acceleration)
  steer/1 -> Steer Safety/1(steering), Brake Safety/4(steering)
  [steeringCommand] -> MATLAB Function5/3(steering)
  Steer Safety/1(actualSteeringCommand) -> actualSteeringCommand/1
  [flag] -> Brake Safety/2(flag), Steer Safety/2(flag), MATLAB Function5/5(flag)
  deceleration/1 -> Brake Safety/1(deceleration)
  [egoVelocity] -> MATLAB Function5/4(velocity)
  MATLAB Function5/1(stopSimFlag) -> stopSimFlag/1
  velocity/1 -> Brake Safety/3(velocity)

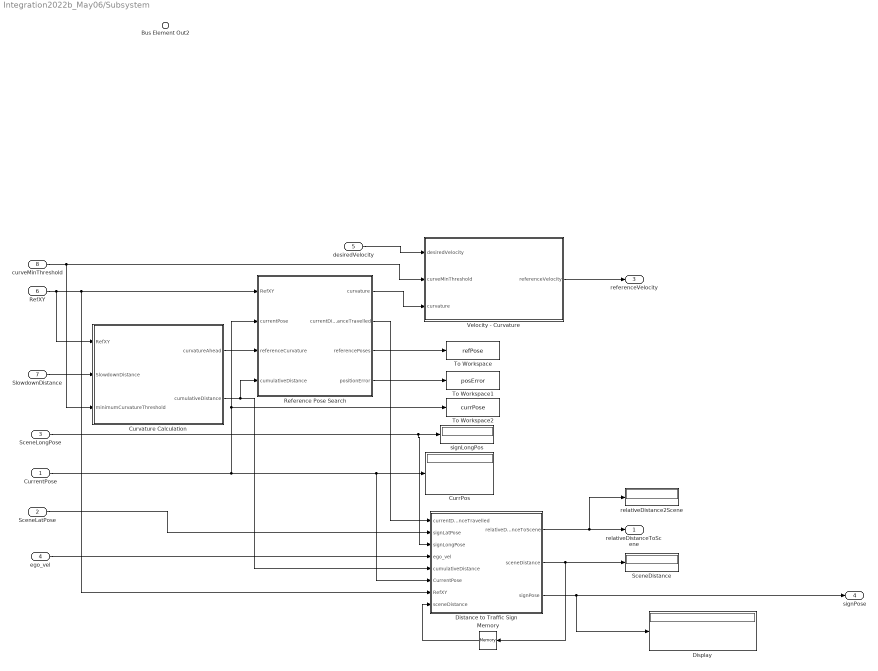
== system Integration2022b_May06/Subsystem ==
  CurrentPose : Inport
  SceneLatPose : Inport  Port=2
  SceneLongPose : Inport  Port=3
  ego_vel : Inport  Port=4
  desiredVelocity : Inport  Port=5
  RefXY : Inport  Port=6
  SlowdownDistance : Inport  Port=7
  curveMinThreshold : Inport  Port=8
  CurrPos : Display
  Curvature Calculation : MATLAB Function  TreatAsAtomicUnit=on
  Display : Display
  Distance to Traffic Sign : MATLAB Function  TreatAsAtomicUnit=on
  Memory : Memory  InitialCondition=40
  Reference Pose Search : MATLAB Function  TreatAsAtomicUnit=on
  SceneDistance : Display
  To Workspace : ToWorkspace  VariableName=refPose  SaveFormat=Structure  SampleTime=-1
      settings: Save2DSignal=2-D array (concatenate along first dimension)
  To Workspace1 : ToWorkspace  VariableName=posError  SaveFormat=Structure  SampleTime=-1
      settings: Save2DSignal=2-D array (concatenate along first dimension)
  To Workspace2 : ToWorkspace  VariableName=currPose  SaveFormat=Structure  SampleTime=-1
      settings: Save2DSignal=2-D array (concatenate along first dimension)
  Velocity - Curvature : MATLAB Function  TreatAsAtomicUnit=on
  relativeDistance2Scene : Display
  signLongPos : Display
  relativeDistanceToScene : Outport
  Bus Element Out2 : Outport  Port=2  PortName=OutBus  Element=signal1
  referenceVelocity : Outport  Port=3
  signPose : Outport  Port=4
  wires:
  Distance to Traffic Sign/3(signPose) -> Display/1, signPose/1
  Distance to Traffic Sign/2(sceneDistance) -> SceneDistance/1, Memory/1
  Distance to Traffic Sign/1(relativeDistanceToScene) -> relativeDistanceToScene/1, relativeDistance2Scene/1
  Velocity - Curvature/1(referenceVelocity) -> referenceVelocity/1
  ego_vel/1 -> Distance to Traffic Sign/4(ego_vel)
  RefXY/1 -> Distance to Traffic Sign/7(RefXY), Reference Pose Search/1(RefXY), Curvature Calculation/1(RefXY)
  CurrentPose/1 -> To Workspace2/1, Reference Pose Search/2(currentPose), Distance to Traffic Sign/6(CurrentPose), CurrPos/1
  Curvature Calculation/1(curvatureAhead) -> Reference Pose Search/3(referenceCurvature)
  Memory/1 -> Distance to Traffic Sign/8("sceneDistance ")
  Curvature Calculation/2(cumulativeDistance) -> Reference Pose Search/4(cumulativeDistance), Distance to Traffic Sign/5(cumulativeDistance)
  desiredVelocity/1 -> Velocity - Curvature/1(desiredVelocity)
  Reference Pose Search/1(curvature) -> Velocity - Curvature/3(curvature)
  SceneLongPose/1 -> Distance to Traffic Sign/3(signLongPose), signLongPos/1
  curveMinThreshold/1 -> Curvature Calculation/3(minimumCurvatureThreshold), Velocity - Curvature/2(curveMinThreshold)
  SlowdownDistance/1 -> Curvature Calculation/2(SlowdownDistance)
  Reference Pose Search/2(currentDistanceTravelled) -> Distance to Traffic Sign/1(currentDistanceTravelled)
  SceneLatPose/1 -> Distance to Traffic Sign/2(signLatPose)
  Reference Pose Search/3(referencePoses) -> To Workspace/1
  Reference Pose Search/4(positionError) -> To Workspace1/1

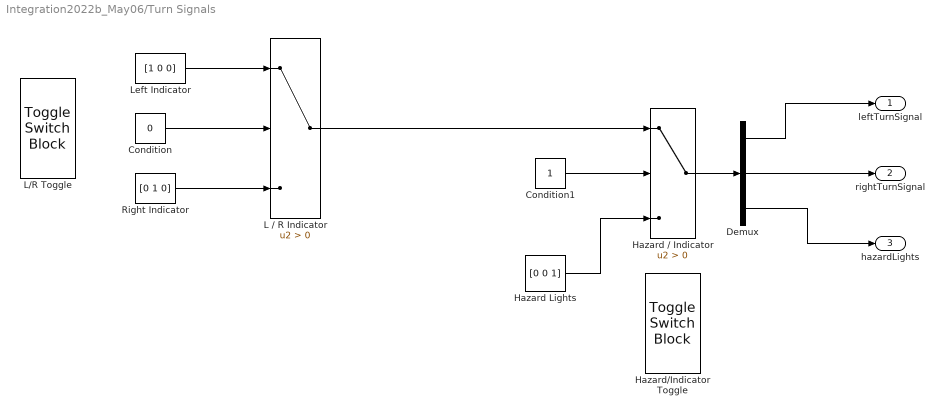
== system Integration2022b_May06/Turn Signals ==
  Condition : Constant  Value=0
  Condition1 : Constant
  Demux : Demux  Outputs=3
  Hazard / Indicator : Switch  Criteria=u2 > Threshold  SaturateOnIntegerOverflow=off  InputSameDT=off
  Hazard Lights : Constant  Value=[0 0 1]
  Hazard/Indicator Toggle : ToggleSwitchBlock
      settings: Values={{'Off', 'On'}, [0 1]}
  L / R Indicator : Switch  Criteria=u2 > Threshold  SaturateOnIntegerOverflow=off  InputSameDT=off
  L/R Toggle : ToggleSwitchBlock
      settings: Values={{'Off', 'On'}, [0 1]}
  Left Indicator : Constant  Value=[1 0 0]
  Right Indicator : Constant  Value=[0 1 0]
  leftTurnSignal : Outport
  rightTurnSignal : Outport  Port=2
  hazardLights : Outport  Port=3
  wires:
  Left Indicator/1 -> L / R Indicator/1
  Condition/1 -> L / R Indicator/2
  Condition1/1 -> Hazard / Indicator/2
  Right Indicator/1 -> L / R Indicator/3
  Hazard Lights/1 -> Hazard / Indicator/3
  L / R Indicator/1 -> Hazard / Indicator/1
  Demux/1 -> leftTurnSignal/1
  Demux/2 -> rightTurnSignal/1
  Demux/3 -> hazardLights/1
  Hazard / Indicator/1 -> Demux/1

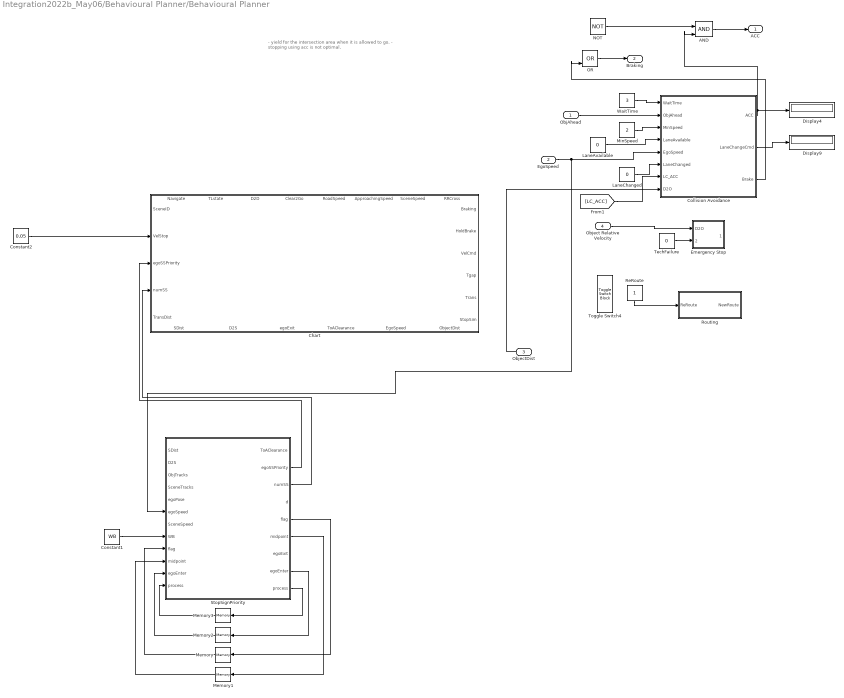
== system Integration2022b_May06/Behavioural Planner/Behavioural Planner ==
  note: - yield for the intersection area when it is allowed to go.
      | - stopping using acc is not optimal.
  ObjAhead : Inport
  EgoSpeed : Inport  Port=2
  ObjectDist : Inport  Port=3
  Object Relative Velocity : Inport  Port=4
  AND : Logic  IconShape=distinctive  AllPortsSameDT=off  OutDataTypeStr=fixdt(1,16)
  Chart : Stateflow chart  TreatAsAtomicUnit=on
      settings: PortSchema="{\"entries\":[{\"content\":{\"sides\":[{\"content\":{\"connectorIds\":[\"In17\",\"In18\",\"In19\",\"In2\",\"In5\"]},\"type\":\"ConnectorPlacement.EquallySpacedRectSide\",\"uuid\":\"81aca70f-0947-49fb-b60a-be241e44193b\"},{\"content\":{\"connectorIds\":[\"Out6\",\"Out2\",\"Out1\",\"Out3\",\"Out4\",\"Out5\"],\"side\":\"RIGHT\"},\"type\":\"ConnectorPlacement.EquallySpacedRectSide\",\"uuid\":\"e7b9645e-3711-4964-ac9b-0199dd335e99\"},{\"content\":{\"connectorIds\":[\"In13\",\"In1\",\"In14\",\"In15\",\"In16\",\"In6\",\"In9\",\"In11\"],\"side\":\"TOP\"},\"type\":\"ConnectorPlacement.EquallySpacedRectSide\",\"uuid\":\"6876f024-944b-4540-9404-d68f37763657\"},{\"content\":{\"connectorIds\":[\"In10\",\"In12\",\"In3\",\"In4\",\"In7\",\"In8\"],\"side\":\"BOTTOM\"},\"type\":\"ConnectorPlacement.EquallySpacedRectSide\",\"uuid\":\"44acab73-cdde-4edf-95df-27422644ccab\"}]},\"type\":\"ConnectorPlacement.EquallySpacedConnector\",\"uuid\":\"d2c31c01-e447-43db-8d2b-8b98a0ca291a\"}],\"packageUris\":[\"http://schema.mathworks.com/mf0/Connector/R2020b\"],\"version\":\"1.0\"}"
  Collision Avoidance : Stateflow chart  TreatAsAtomicUnit=on
  Constant1 : Constant  Value=WB
  Constant2 : Constant  Value=0.05
  Display4 : Display
  Display9 : Display
  Emergency Stop : Stateflow chart  TreatAsAtomicUnit=on
  LaneAvailable : Constant  Value=0
  LaneChanged : Constant  Value=0
  Memory : Memory
  Memory1 : Memory  InitialCondition=[0 0]
  Memory2 : Memory
  Memory3 : Memory  InitialCondition=1
  MinSpeed : Constant  Value=2
  NOT : Logic  Operator=NOT  IconShape=distinctive  AllPortsSameDT=off  OutDataTypeStr=boolean
  OR : Logic  Operator=OR  IconShape=distinctive  AllPortsSameDT=off  OutDataTypeStr=boolean
  ReRoute : Constant
  Routing : Stateflow chart  TreatAsAtomicUnit=on
  StopSignPriority : MATLAB Function  TreatAsAtomicUnit=on
  TechFailure : Constant  Value=0
  Toggle Switch4 : ToggleSwitchBlock
      settings: Values={{'Off', 'On'}, [0 1]}
  WaitTime : Constant  Value=3
  ACC : Outport
  Braking : Outport  Port=2
  wires:
  ObjectDist/1 -> Collision Avoidance/8(D2O)
  WaitTime/1 -> Collision Avoidance/1(WaitTime)
  EgoSpeed/1 -> Collision Avoidance/5(EgoSpeed), StopSignPriority/6(egoSpeed)
  ReRoute/1 -> Routing/1(ReRoute)
  Collision Avoidance/2(LaneChangeCmd) -> Display9/1
  LaneAvailable/1 -> Collision Avoidance/4(LaneAvailable)
  MinSpeed/1 -> Collision Avoidance/3(MinSpeed)
  LaneChanged/1 -> Collision Avoidance/6(LaneChanged)
  ObjAhead/1 -> Collision Avoidance/2(ObjAhead)
  TechFailure/1 -> Emergency Stop/2(TechFailure)
  Object Relative Velocity/1 -> Emergency Stop/1(D2O)
  Collision Avoidance/1(ACC) -> AND/2, Display4/1
  NOT/1 -> AND/1
  AND/1 -> ACC/1
  OR/1 -> Braking/1
  Collision Avoidance/3(Brake) -> OR/2
  [LC_ACC] -> Collision Avoidance/7(LC_ACC)
  Constant2/1 -> Chart/18(VelStop)
  StopSignPriority/2(egoSSPriority) -> Chart/19(egoSSPriority)
  StopSignPriority/3(numSS) -> Chart/2(numSS)
  Constant1/1 -> StopSignPriority/8(WB)
  Memory/1 -> StopSignPriority/9("flag ")
  StopSignPriority/5(flag) -> Memory/1
  StopSignPriority/6(midpoint) -> Memory1/1
  Memory1/1 -> StopSignPriority/10("midpoint ")
  StopSignPriority/8(egoEnter) -> Memory2/1
  Memory2/1 -> StopSignPriority/11("egoEnter ")
  StopSignPriority/9(process) -> Memory3/1
  Memory3/1 -> StopSignPriority/12("process ")

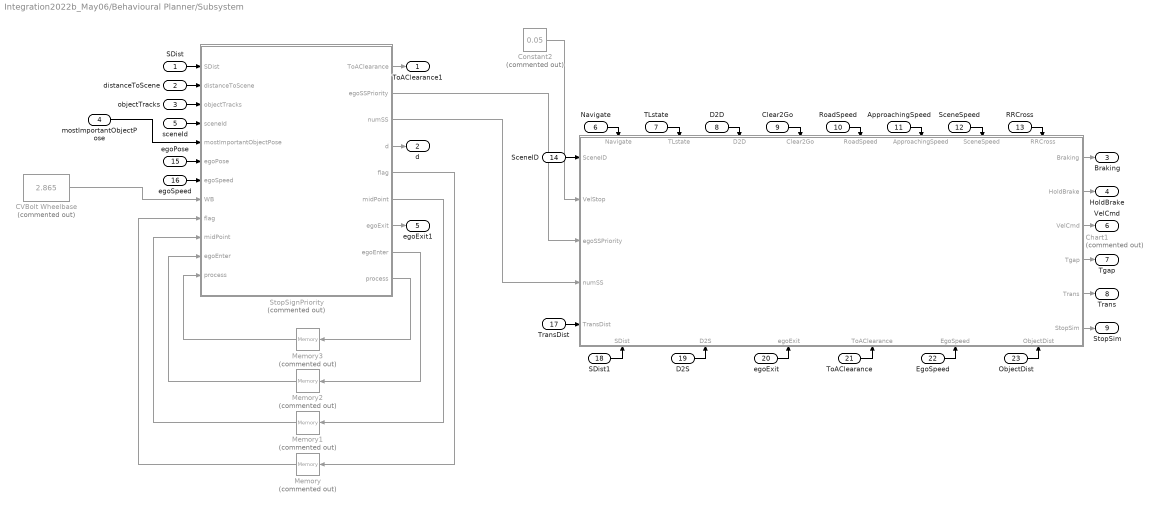
== system Integration2022b_May06/Behavioural Planner/Subsystem ==
  SDist : Inport
  distanceToScene : Inport  Port=2
  objectTracks : Inport  Port=3
  mostImportantObjectPose : Inport  Port=4
  sceneId : Inport  Port=5
  Navigate : Inport  Port=6
  TLstate : Inport  Port=7
  D2D : Inport  Port=8
  Clear2Go : Inport  Port=9
  RoadSpeed : Inport  Port=10
  ApproachingSpeed : Inport  Port=11
  SceneSpeed : Inport  Port=12
  RRCross : Inport  Port=13
  SceneID : Inport  Port=14
  egoPose : Inport  Port=15
  egoSpeed : Inport  Port=16
  TransDist : Inport  Port=17
  SDist1 : Inport  Port=18
  D2S : Inport  Port=19
  egoExit : Inport  Port=20
  ToAClearance : Inport  Port=21
  EgoSpeed : Inport  Port=22
  ObjectDist : Inport  Port=23
  CVBolt Wheelbase : Constant  Commented=on  Value=2.865
  Chart1 : Stateflow chart  Commented=on  TreatAsAtomicUnit=on
      settings: PortSchema="{\"entries\":[{\"content\":{\"sides\":[{\"content\":{\"connectorIds\":[\"In17\",\"In18\",\"In19\",\"In2\",\"In5\"]},\"type\":\"ConnectorPlacement.EquallySpacedRectSide\",\"uuid\":\"81aca70f-0947-49fb-b60a-be241e44193b\"},{\"content\":{\"connectorIds\":[\"Out6\",\"Out2\",\"Out1\",\"Out3\",\"Out4\",\"Out5\"],\"side\":\"RIGHT\"},\"type\":\"ConnectorPlacement.EquallySpacedRectSide\",\"uuid\":\"e7b9645e-3711-4964-ac9b-0199dd335e99\"},{\"content\":{\"connectorIds\":[\"In13\",\"In1\",\"In14\",\"In15\",\"In16\",\"In6\",\"In9\",\"In11\"],\"side\":\"TOP\"},\"type\":\"ConnectorPlacement.EquallySpacedRectSide\",\"uuid\":\"6876f024-944b-4540-9404-d68f37763657\"},{\"content\":{\"connectorIds\":[\"In10\",\"In12\",\"In3\",\"In4\",\"In7\",\"In8\"],\"side\":\"BOTTOM\"},\"type\":\"ConnectorPlacement.EquallySpacedRectSide\",\"uuid\":\"44acab73-cdde-4edf-95df-27422644ccab\"}]},\"type\":\"ConnectorPlacement.EquallySpacedConnector\",\"uuid\":\"d2c31c01-e447-43db-8d2b-8b98a0ca291a\"}],\"packageUris\":[\"http://schema.mathworks.com/mf0/Connector/R2020b\"],\"version\":\"1.0\"}"
  Constant2 : Constant  Commented=on  Value=0.05
  Memory : Memory  Commented=on
  Memory1 : Memory  Commented=on  InitialCondition=[0 0]
  Memory2 : Memory  Commented=on
  Memory3 : Memory  Commented=on  InitialCondition=1
  StopSignPriority : MATLAB Function  Commented=on  TreatAsAtomicUnit=on
  ToAClearance1 : Outport
  d : Outport  Port=2
  Braking : Outport  Port=3
  HoldBrake : Outport  Port=4
  egoExit1 : Outport  Port=5
  VelCmd : Outport  Port=6
  Tgap : Outport  Port=7
  Trans : Outport  Port=8
  StopSim : Outport  Port=9
  wires:
  egoSpeed/1 -> StopSignPriority/7(egoSpeed)
  Memory1/1 -> StopSignPriority/10("midPoint ")
  Memory/1 -> StopSignPriority/9("flag ")
  distanceToScene/1 -> StopSignPriority/2(distanceToScene)
  objectTracks/1 -> StopSignPriority/3(objectTracks)
  Constant2/1 -> Chart1/18(VelStop)
  mostImportantObjectPose/1 -> StopSignPriority/5(mostImportantObjectPose)
  Chart1/3(Tgap) -> Tgap/1
  StopSignPriority/9(process) -> Memory3/1
  SceneSpeed/1 -> Chart1/9(SceneSpeed)
  StopSignPriority/3(numSS) -> Chart1/2(numSS)
  Chart1/6(Braking) -> Braking/1
  Memory2/1 -> StopSignPriority/11("egoEnter ")
  StopSignPriority/8(egoEnter) -> Memory2/1
  Memory3/1 -> StopSignPriority/12("process ")
  ToAClearance/1 -> Chart1/4(ToAClearance)
  StopSignPriority/5(flag) -> Memory/1
  sceneId/1 -> StopSignPriority/4(sceneId)
  StopSignPriority/2(egoSSPriority) -> Chart1/19(egoSSPriority)
  Chart1/4(Trans) -> Trans/1
  TLstate/1 -> Chart1/1(TLstate)
  StopSignPriority/1(ToAClearance) -> ToAClearance1/1
  StopSignPriority/6(midPoint) -> Memory1/1
  CVBolt Wheelbase/1 -> StopSignPriority/8(WB)
  ApproachingSpeed/1 -> Chart1/6(ApproachingSpeed)
  StopSignPriority/4(d) -> d/1
  EgoSpeed/1 -> Chart1/7(EgoSpeed)
  D2D/1 -> Chart1/14(D2D)
  Clear2Go/1 -> Chart1/15(Clear2Go)
  egoExit/1 -> Chart1/3(egoExit)
  TransDist/1 -> Chart1/5(TransDist)
  RoadSpeed/1 -> Chart1/16(RoadSpeed)
  Chart1/2(HoldBrake) -> HoldBrake/1
  StopSignPriority/7(egoExit) -> egoExit1/1
  SceneID/1 -> Chart1/17(SceneID)
  egoPose/1 -> StopSignPriority/6(egoPose)
  Chart1/5(StopSim) -> StopSim/1
  Chart1/1(VelCmd) -> VelCmd/1
  Navigate/1 -> Chart1/13(Navigate)
  RRCross/1 -> Chart1/11(RRCross)
  SDist1/1 -> Chart1/10(SDist)
  SDist/1 -> StopSignPriority/1(SDist)
  D2S/1 -> Chart1/12(D2S)
  ObjectDist/1 -> Chart1/8(ObjectDist)

== system Integration2022b_May06/Controllers/Lateral Controller ==
  Pose : Inport
  waypoints : Inport  Port=2
  Pure Pursuit Controller1 : Subsystem
  SteeringRatio : Gain  Gain=16
  rad to degree : Gain  Gain=180/pi
  steeringCommand : Outport
  wires:
  Pose/1 -> Pure Pursuit Controller1/1(Pose)
  waypoints/1 -> Pure Pursuit Controller1/2(Waypoints)
  rad to degree/1 -> SteeringRatio/1
  SteeringRatio/1 -> steeringCommand/1
  Pure Pursuit Controller1/1(delta) -> rad to degree/1

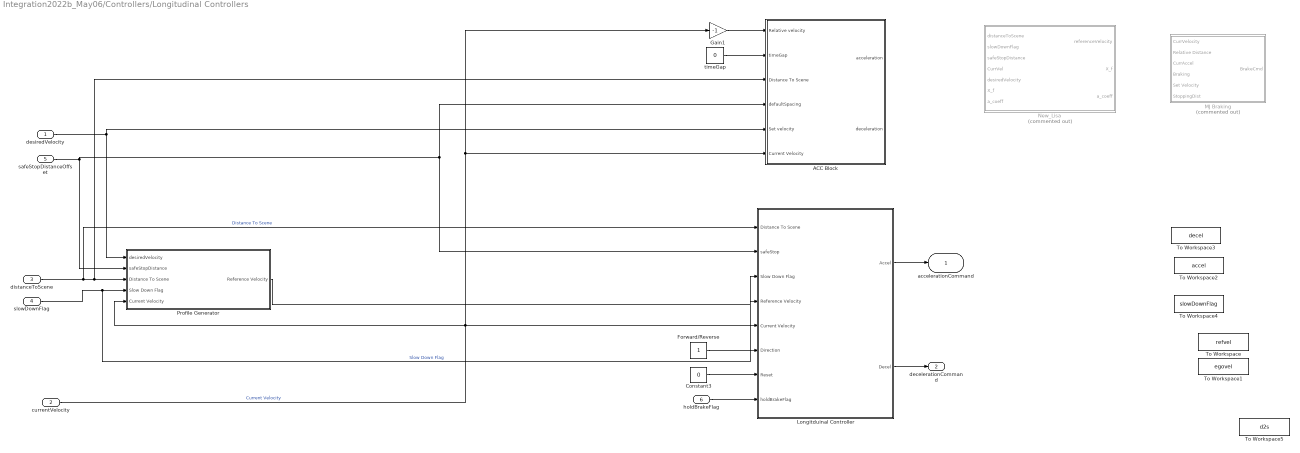
== system Integration2022b_May06/Controllers/Longitudinal Controllers ==
  desiredVelocity : Inport
  currentVelocity : Inport  Port=2
  distanceToScene : Inport  Port=3
  slowDownFlag : Inport  Port=4
  safeStopDistanceOffset : Inport  Port=5
  holdBrakeFlag : Inport  Port=6
  ACC Block : Subsystem
  Constant3 : Constant  Value=0
  Forward/Reverse : Constant
  Gain1 : Gain  Gain=-1
  Longitduinal Controller : Subsystem
  MJ Braking : Subsystem  Commented=on
  New_Lisa : MATLAB Function  Commented=on  TreatAsAtomicUnit=on
  Profile Generator : Subsystem
  To Workspace : ToWorkspace  VariableName=refvel  SaveFormat=Structure  SampleTime=-1
      settings: Save2DSignal=2-D array (concatenate along first dimension)
  To Workspace1 : ToWorkspace  VariableName=egovel  SaveFormat=Structure  SampleTime=-1
      settings: Save2DSignal=2-D array (concatenate along first dimension)
  To Workspace2 : ToWorkspace  VariableName=accel  SaveFormat=Structure  SampleTime=-1
      settings: Save2DSignal=2-D array (concatenate along first dimension)
  To Workspace3 : ToWorkspace  VariableName=decel  SaveFormat=Structure  SampleTime=-1
      settings: Save2DSignal=2-D array (concatenate along first dimension)
  To Workspace4 : ToWorkspace  VariableName=slowDownFlag  SaveFormat=Structure  SampleTime=-1
      settings: Save2DSignal=2-D array (concatenate along first dimension)
  To Workspace5 : ToWorkspace  VariableName=d2s  SaveFormat=Structure  SampleTime=-1
      settings: Save2DSignal=2-D array (concatenate along first dimension)
  timeGap : Constant  Value=0
  accelerationCommand : Outport
  decelerationCommand : Outport  Port=2
  wires:
  distanceToScene/1 -> Longitduinal Controller/1(Distance To Scene), ACC Block/3(Distance To Scene), Profile Generator/3(Distance To Scene)  "Distance To Scene"
  slowDownFlag/1 -> Profile Generator/4(Slow Down Flag), Longitduinal Controller/3(Slow Down Flag)  "Slow Down Flag"
  currentVelocity/1 -> Profile Generator/5(Current Velocity), ACC Block/6(Current Velocity), Gain1/1, Longitduinal Controller/5(Current Velocity)  "Current Velocity"
  safeStopDistanceOffset/1 -> ACC Block/4(defaultSpacing), Longitduinal Controller/2(safeStop), Profile Generator/2(safeStopDistance)
  Gain1/1 -> ACC Block/1(Relative velocity)
  timeGap/1 -> ACC Block/2(timeGap)
  desiredVelocity/1 -> ACC Block/5(Set velocity), Profile Generator/1(desiredVelocity)
  Forward/Reverse/1 -> Longitduinal Controller/6(Direction)
  Constant3/1 -> Longitduinal Controller/7(Reset)
  holdBrakeFlag/1 -> Longitduinal Controller/8(holdBrakeFlag)
  Longitduinal Controller/1(Accel) -> accelerationCommand/1
  Longitduinal Controller/2(Decel) -> decelerationCommand/1
  Profile Generator/1(Reference Velocity) -> Longitduinal Controller/4(Reference Velocity)
